simulink model "Test_Encoder_16_to_4"  (Simulink 8.7)
settings: Solver=ode45  StartTime=0.0  StopTime=len  RelTol=1e-3
libraries: commutil2 x2, Encoders_Lib x1
settings Model: Creator=N  LastModifiedBy=Jozko Mrkvicka
settings DataIOCC: LimitDataPoints=off
settings DebuggingCC: UnderspecifiedInitializationDetection=Simplified  MergeDetectMultiDrivingBlocksExec=error
settings HardwareCC: ProdBitPerPointer=64  ProdLargestAtomicFloat=Float  ProdIntDivRoundTo=Zero  ProdEndianess=LittleEndian  ProdHWDeviceType=Intel->x86-64 (Windows64)
settings ModelReferenceCC: PropagateSignalLabelsOutOfModel=on

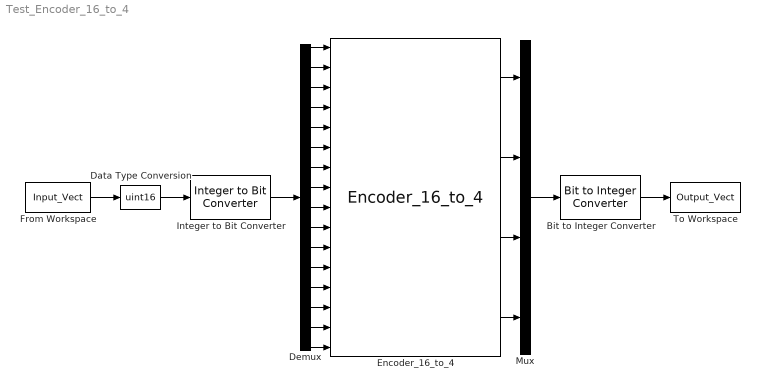
== system Test_Encoder_16_to_4 ==
  Bit to Integer Converter : commutil2/Bit to Integer Converter  nbits=4  bitOrder=MSB first  signedOutputValues=Unsigned  outDtype=uint16  outDtypeSigned=Inherit via internal rule
  Data Type Conversion : DataTypeConversion  OutDataTypeStr=uint16
  Demux : Demux  Outputs=16
  Encoder_16_to_4 : Encoders_Lib/Encoders_Lib/Encoder_16_to_4
  From Workspace : FromWorkspace  VariableName=Input_Vect  SampleTime=1  Interpolate=off  OutputAfterFinalValue=Holding final value
  Integer to Bit Converter : commutil2/Integer to Bit Converter  nbits=16  signedInputValues=Unsigned  bitOrder=MSB first  outDtype=boolean
  Mux : Mux
  To Workspace : ToWorkspace  VariableName=Output_Vect  SampleTime=1
  wires:
  Demux/1 -> Encoder_16_to_4/1
  Demux/2 -> Encoder_16_to_4/2
  Demux/3 -> Encoder_16_to_4/3
  Demux/4 -> Encoder_16_to_4/4
  Demux/5 -> Encoder_16_to_4/5
  Demux/7 -> Encoder_16_to_4/7
  Demux/8 -> Encoder_16_to_4/8
  Demux/6 -> Encoder_16_to_4/6
  Demux/9 -> Encoder_16_to_4/9
  Demux/10 -> Encoder_16_to_4/10
  Demux/11 -> Encoder_16_to_4/11
  Demux/12 -> Encoder_16_to_4/12
  Demux/13 -> Encoder_16_to_4/13
  Demux/14 -> Encoder_16_to_4/14
  Demux/15 -> Encoder_16_to_4/15
  Demux/16 -> Encoder_16_to_4/16
  Encoder_16_to_4/1 -> Mux/1
  Encoder_16_to_4/4 -> Mux/4
  Encoder_16_to_4/3 -> Mux/3
  Encoder_16_to_4/2 -> Mux/2
  Mux/1 -> Bit to Integer Converter/1
  Bit to Integer Converter/1 -> To Workspace/1
  Integer to Bit Converter/1 -> Demux/1
  Data Type Conversion/1 -> Integer to Bit Converter/1
  From Workspace/1 -> Data Type Conversion/1
